simulink model "Fuzzy_manobra_aplicado_2015b"  (R2015b)
settings: Solver=ode1  StartTime=0.0  StopTime=t_final  FixedStep=0.01  RelTol=1e-3
values from neighbouring files (symbols this model uses):
  fis = readfis(['CONTROLADORES/' controlador '.fis'])    [inicia_fuzzy_manobra.m]
  k_i = 1    [inicia_fuzzy_manobra.m]
  k_p = 2.5    [inicia_fuzzy_manobra.m]
  L = 0.1175    [inicia_fuzzy_manobra.m]
  N_sp = size(setpoints,1)    [inicia_fuzzy_manobra.m]
  R = 0.034    [inicia_fuzzy_manobra.m]
undefined symbols (not defined in the file or in its folder): HIL, magnitude, setpoints
libraries: quarc_library x6, simulink x3, fuzblock x1
settings Model: SimulationMode=external  ExtModeTrigDuration=10000  Creator=rhuq  LastModifiedBy=LabMTrônica01
settings SolverCC: PositivePriorityOrder=on
settings DataIOCC: LimitDataPoints=off  SaveFormat=Array  SignalLoggingSaveFormat=ModelDataLogs
settings OptimizationCC: ExpressionDepthLimit=2147483647  InitFltsAndDblsToZero=on
settings DebuggingCC: SaveWithParameterizedLinksMsg=none  UnderspecifiedInitializationDetection=Classic  MergeDetectMultiDrivingBlocksExec=none  SolverPrmCheckMsg=warning  ParameterPrecisionLossMsg=none  FcnCallInpInsideContextMsg=EnableAllAsWarning  StateNameClashWarn=warning
settings HardwareCC: ProdBitPerPointer=32  ProdLargestAtomicFloat=None  ProdIntDivRoundTo=Undefined  ProdEndianess=Unspecified  ProdWordSize=32  ProdHWDeviceType=32-bit Generic
settings SFSimCC: SimParseCustomCode=off
settings RTWCC: SystemTargetFile=quarc_linux_duovero.tlc  TemplateMakefile=quarc_default_tmf  Description=QUARC Linux DuoVero Target
settings STFCustomTargetCC: TargetLibSuffix=.a  TargetPreCompLibLocation=C:\PROGRA~3\QUARC\lib\2015b\LINUX_~1\release  GeneratePreprocessorConditionals=Use local settings  CombineOutputUpdateFcns=on  GRTInterface=off  SystemTargetFile=quarc_linux_duovero.tlc
settings GRTTargetCC: TargetLibSuffix=.a  TargetPreCompLibLocation=C:\PROGRA~3\QUARC\lib\2015b\LINUX_~1\release  ParMdlRefBuildCompliant=off  CompOptLevelCompliant=off  MatFileLogging=off  UseToolchainInfoCompliant=off  ExtMode=on  ExtModeMexFile=quarc_comm  ExtModeMexArgs='-w -d /tmp -uri %u'
settings ConfigComp: CovModelRefEnable=Off

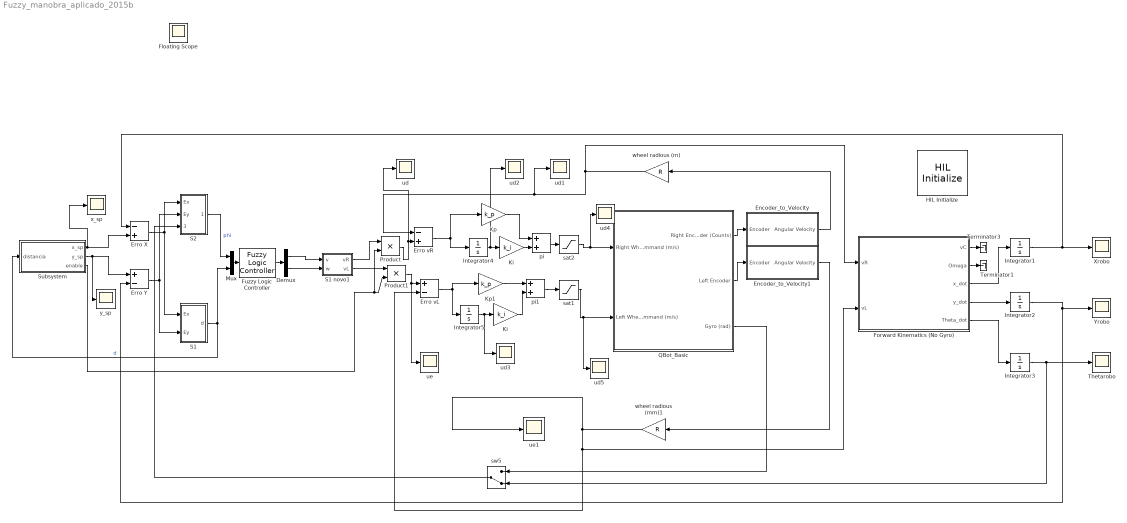
== system Fuzzy_manobra_aplicado_2015b ==
  Demux : Demux  Outputs=2
  Encoder_to_Velocity : Subsystem
  Encoder_to_Velocity1 : Subsystem
  Erro X : Sum  Inputs=-+
  Erro Y : Sum  Inputs=+-
  Erro vL : Sum  Inputs=+-
  Erro vR : Sum  Inputs=-+
  Forward Kinematics (No Gyro) : Subsystem
  Fuzzy Logic Controller : fuzblock/Fuzzy Logic  Controller  fis=[fis]
  HIL Initialize : quarc_library/Data Acquisition/Generic/Configuration/HIL Initialize  Priority=-99  object_name=HIL-1  board_type=qbot2  board_number=0  board_options=enc0_dir=0;enc0_filter=1;enc0_a=0;enc0_b=0;enc0_z=1;enc0_reload=0;enc1_dir=0;enc1_filter=1;enc1_a=0;enc1_b=0;enc1_z=1;enc1_reload=0;pwm0_immediate=0;pwm1_immediate=0;pwm2_immediate=0;pwm3_immediate=0;  exclusive=off  active=off  hardware_clocks=[]  clock_modes=[]  initial_clock_frequencies=[]  set_clock_params_at_start=off  set_clock_params_at_switch_in=off  set_clock_frequencies_at_start=off  set_clock_frequencies_at_switch_in=off  analog_input_channels=[0:9]  analog_input_maximums=[5 5 5 5 16.5 3.3 3.3 3.3 3.3]  analog_input_minimums=[0 0 0 0 0 0 0 0 0]  set_analog_input_params_at_start=off  set_analog_input_params_at_switch_in=off  analog_output_channels=[]  analog_output_maximums=[]  analog_output_minimums=[]  initial_analog_outputs=[]  final_analog_outputs=[]  watchdog_analog_outputs=[]  set_analog_output_params_at_start=off  set_analog_output_params_at_switch_in=off  set_analog_outputs_at_start=off  set_analog_outputs_at_switch_in=off  set_analog_outputs_at_terminate=off  set_analog_outputs_at_switch_out=off  set_analog_outputs_on_watchdog=off  digital_input_channels=[]  digital_output_channels=[]  digital_output_configuration=[]  initial_digital_outputs=[0]  final_digital_outputs=[0]  watchdog_digital_outputs=[0]  set_digital_output_params_at_start=off  set_digital_output_params_at_switch_in=off  set_digital_outputs_at_start=on  set_digital_outputs_at_switch_in=off  set_digital_outputs_at_terminate=on  set_digital_outputs_at_switch_out=off  set_digital_outputs_on_watchdog=on  encoder_channels=[0:3]  quadrature=[4]  encoder_filter_frequency=[]  initial_encoder_counts=[0]  set_encoder_params_at_start=on  set_encoder_params_at_switch_in=off  set_encoder_counts_at_start=on  set_encoder_counts_at_switch_in=off  pwm_channels=[0:3]  pwm_modes=[0 0 0 0]  pwm_frequency=[20e6/1024 20e6/1024 20e6/1024 20e6/1024]  pwm_configuration=[0]  pwm_alignment=[0]  pwm_polarity=[1]  pwm_leading_deadband=[0]  pwm_trailing_deadband=[0]  initial_pwm_outputs=[0]  final_pwm_outputs=[0]  watchdog_pwm_outputs=[0]  set_pwm_params_at_start=on  set_pwm_params_at_switch_in=off  set_pwm_outputs_at_start=on  set_pwm_outputs_at_switch_in=off  set_pwm_outputs_at_terminate=on  set_pwm_outputs_at_switch_out=off  set_pwm_outputs_on_watchdog=on  other_output_channels=[2000:2001]  initial_other_outputs=[0 0 7]  final_other_outputs=[0 0 1]  watchdog_other_outputs=[]  set_other_outputs_at_start=on  set_other_outputs_at_switch_in=off  set_other_outputs_at_terminate=on  set_other_outputs_at_switch_out=off  set_other_outputs_on_watchdog=off
  Integrator1 : Integrator  ContinuousStateAttributes='x_a'
  Integrator2 : Integrator  ContinuousStateAttributes='y_a'
  Integrator3 : Integrator  ContinuousStateAttributes='theta'
  Integrator4 : Integrator  ContinuousStateAttributes='ePI_d'
  Integrator5 : Integrator  ContinuousStateAttributes='ePI_e'
  Ki : Gain  Gain=k_i
  "Ki " : Gain  Gain=k_i
  Kp : Gain  Gain=k_p
  Kp1 : Gain  Gain=k_p
  Mux : Mux  Inputs=2
  Product : Product
  Product1 : Product
  QBot_Basic : Subsystem
  S1 : Subsystem
  S1 novo1 : Subsystem
  S2 : Subsystem
  Subsystem : Subsystem
  Terminator1 : Terminator
  Terminator3 : Terminator
  Thetarobo : Scope
  Xrobo : Scope
  Yrobo : Scope
  pi : Sum
  pi1 : Sum
  sat1 : Saturate  UpperLimit=0.65  LowerLimit=-0.65
  sat2 : Saturate  UpperLimit=0.65  LowerLimit=-0.65
  sw5 : ManualSwitch  CurrentSetting=0
  ud{,1..5} (6 alike) : Scope
  ue : Scope
  ue1 : Scope
  wheel radious (m) : Gain  Gain=R
  wheel radious (mm)1 : Gain  Gain=R
  x_sp : Scope
  y_sp : Scope
  Floating Scope : Scope
  wires:
  QBot_Basic/1(Right Encoder (Counts)) -> Encoder_to_Velocity/1(Encoder)
  QBot_Basic/2(Left Encoder) -> Encoder_to_Velocity1/1(Encoder)
  Erro X/1 -> S1/1(Ex), S2/1(Ex)
  Erro Y/1 -> S1/2(Ey), S2/2(Ey)
  Mux/1 -> Fuzzy Logic Controller/1
  S2/1(phi) -> Mux/1  "phi"
  Subsystem/2(y_sp) -> Erro Y/1, y_sp/1
  Subsystem/1(x_sp) -> x_sp/1, Erro X/2
  Fuzzy Logic Controller/1 -> Demux/1
  S1 novo1/2(vL) -> Product1/1
  Encoder_to_Velocity1/1(Angular Velocity) -> wheel radious (mm)1/1
  Integrator2/1 -> Yrobo/1, Erro Y/2
  S1/1(d) -> Mux/2, Subsystem/1("distancia ")  "d"
  Demux/1 -> S1 novo1/1(v)
  Demux/2 -> S1 novo1/2(w)
  Encoder_to_Velocity/1(Angular Velocity) -> wheel radious (m)/1
  Forward Kinematics (No Gyro)/3(x_dot) -> Integrator1/1
  Forward Kinematics (No Gyro)/4(y_dot) -> Integrator2/1
  Forward Kinematics (No Gyro)/5(Theta_dot) -> Integrator3/1
  Integrator1/1 -> Xrobo/1, Erro X/1
  Integrator3/1 -> Thetarobo/1, sw5/2
  wheel radious (m)/1 -> ud1/1, Erro vR/1, Forward Kinematics (No Gyro)/1(vR)
  wheel radious (mm)1/1 -> Erro vL/2, Forward Kinematics (No Gyro)/2(vL), ue1/1
  Erro vR/1 -> Kp/1, Integrator4/1
  sw5/1 -> S2/3(theta)
  QBot_Basic/3(Gyro (rad)) -> sw5/1
  Subsystem/3(enable) -> Product/2, Product1/2
  S1 novo1/1(vR) -> Product/1
  Product/1 -> ud/1, Erro vR/2
  sat1/1 -> ud5/1, QBot_Basic/2(Left Wheel Command (m/s))
  sat2/1 -> ud4/1, QBot_Basic/1(Right Wheel Command (m/s))
  Forward Kinematics (No Gyro)/1(vC) -> Terminator3/1
  Forward Kinematics (No Gyro)/2(Omega) -> Terminator1/1
  Erro vL/1 -> Kp1/1, Integrator5/1
  Integrator5/1 -> ud3/1, Ki/1
  Integrator4/1 -> ud2/1, "Ki "/1
  pi1/1 -> sat1/1
  "Ki "/1 -> pi/2
  pi/1 -> sat2/1
  Kp/1 -> pi/1
  Kp1/1 -> pi1/1
  Ki/1 -> pi1/2
  Product1/1 -> ue/1, Erro vL/1

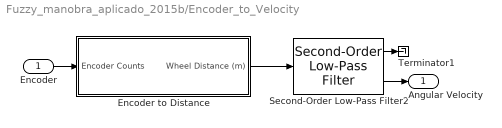
== system Fuzzy_manobra_aplicado_2015b/Encoder_to_Velocity ==
  Encoder : Inport
  Encoder to Distance : Subsystem
  Second-Order Low-Pass Filter2 : quarc_library/Continuous/Second-Order Low-Pass Filter  params_source=Internal (dialog parameters)  input_width=10  input_zeta=1  input_init=0
  Terminator1 : Terminator
  Angular Velocity : Outport
  wires:
  Second-Order Low-Pass Filter2/2 -> Angular Velocity/1
  Encoder/1 -> Encoder to Distance/1(Encoder Counts)
  Encoder to Distance/1(Wheel Distance (m)) -> Second-Order Low-Pass Filter2/1
  Second-Order Low-Pass Filter2/1 -> Terminator1/1

== system Fuzzy_manobra_aplicado_2015b/Encoder_to_Velocity1 ==
  Encoder : Inport
  Encoder to Distance : Subsystem
  Second-Order Low-Pass Filter2 : quarc_library/Continuous/Second-Order Low-Pass Filter  params_source=Internal (dialog parameters)  input_width=10  input_zeta=1  input_init=0
  Terminator1 : Terminator
  Angular Velocity : Outport
  wires:
  Second-Order Low-Pass Filter2/1 -> Terminator1/1
  Encoder to Distance/1(Wheel Distance (m)) -> Second-Order Low-Pass Filter2/1
  Encoder/1 -> Encoder to Distance/1(Encoder Counts)
  Second-Order Low-Pass Filter2/2 -> Angular Velocity/1

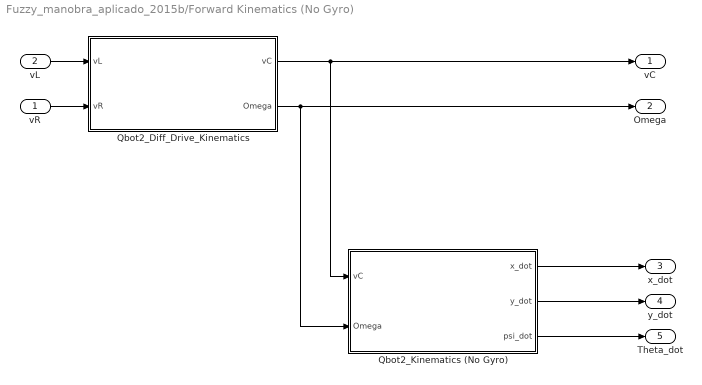
== system Fuzzy_manobra_aplicado_2015b/Forward Kinematics (No Gyro) ==
  vR : Inport
  vL : Inport  Port=2
  Qbot2_Diff_Drive_Kinematics : Subsystem
  Qbot2_Kinematics (No Gyro) : Subsystem
  vC : Outport
  Omega : Outport  Port=2
  x_dot : Outport  Port=3
  y_dot : Outport  Port=4
  Theta_dot : Outport  Port=5
  wires:
  Qbot2_Diff_Drive_Kinematics/2(Omega) -> Qbot2_Kinematics (No Gyro)/2(Omega), Omega/1
  vR/1 -> Qbot2_Diff_Drive_Kinematics/2(vR)
  vL/1 -> Qbot2_Diff_Drive_Kinematics/1(vL)
  Qbot2_Diff_Drive_Kinematics/1(vC) -> Qbot2_Kinematics (No Gyro)/1(vC), vC/1
  Qbot2_Kinematics (No Gyro)/2(y_dot) -> y_dot/1
  Qbot2_Kinematics (No Gyro)/1(x_dot) -> x_dot/1
  Qbot2_Kinematics (No Gyro)/3(psi_dot) -> Theta_dot/1

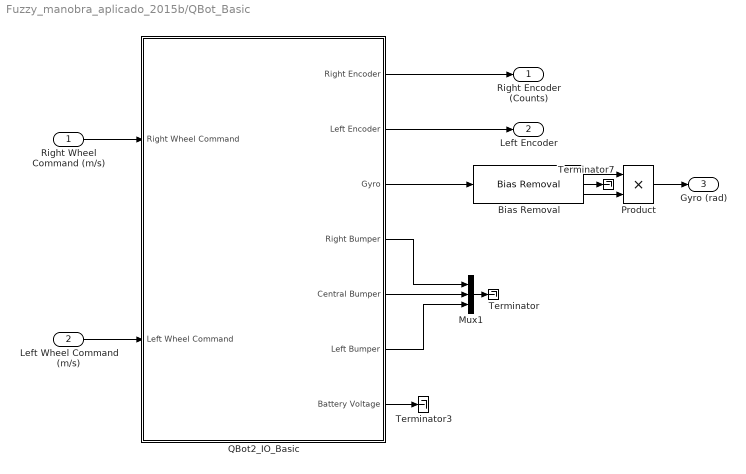
== system Fuzzy_manobra_aplicado_2015b/QBot_Basic ==
  Right Wheel Command (m/s) : Inport
  Left Wheel Command (m/s) : Inport  Port=2
  Bias Removal : quarc_library/Discrete/Bias Removal  start_time=3  end_time=4  switch_id=0  sample_time=qc_get_step_size
  Mux1 : Mux  Inputs=3
  Product : Product  RndMeth=Zero
  QBot2_IO_Basic : Subsystem
  Terminator : Terminator
  Terminator3 : Terminator
  Terminator7 : Terminator
  Right Encoder (Counts) : Outport
  Left Encoder : Outport  Port=2
  Gyro (rad) : Outport  Port=3
  wires:
  Mux1/1 -> Terminator/1
  QBot2_IO_Basic/3(Gyro) -> Bias Removal/1
  Product/1 -> Gyro (rad)/1
  Bias Removal/3 -> Product/2
  Bias Removal/1 -> Product/1
  Bias Removal/2 -> Terminator7/1
  QBot2_IO_Basic/2(Left Encoder) -> Left Encoder/1
  QBot2_IO_Basic/1(Right Encoder) -> Right Encoder (Counts)/1
  Left Wheel Command (m/s)/1 -> QBot2_IO_Basic/2(Left Wheel Command)
  Right Wheel Command (m/s)/1 -> QBot2_IO_Basic/1(Right Wheel Command)
  QBot2_IO_Basic/6(Left Bumper) -> Mux1/3
  QBot2_IO_Basic/5(Central Bumper) -> Mux1/2
  QBot2_IO_Basic/4(Right Bumper) -> Mux1/1
  QBot2_IO_Basic/7(Battery Voltage) -> Terminator3/1

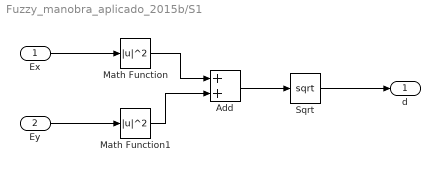
== system Fuzzy_manobra_aplicado_2015b/S1 ==
  Ex : Inport
  Ey : Inport  Port=2
  Add : Sum
  Math Function : Math  Operator=magnitude^2  SaturateOnIntegerOverflow=on
  Math Function1 : Math  Operator=magnitude^2  SaturateOnIntegerOverflow=on
  Sqrt : Sqrt  SaturateOnIntegerOverflow=on
  d : Outport
  wires:
  Math Function/1 -> Add/1
  Ey/1 -> Math Function1/1
  Add/1 -> Sqrt/1
  Ex/1 -> Math Function/1
  Sqrt/1 -> d/1
  Math Function1/1 -> Add/2

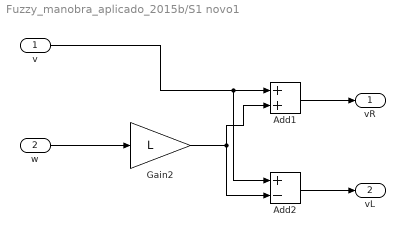
== system Fuzzy_manobra_aplicado_2015b/S1 novo1 ==
  v : Inport
  w : Inport  Port=2
  Add1 : Sum
  Add2 : Sum  Inputs=+-
  Gain2 : Gain  Gain=L
  vR : Outport
  vL : Outport  Port=2
  wires:
  Add1/1 -> vR/1
  v/1 -> Add2/1, Add1/1
  Gain2/1 -> Add1/2, Add2/2
  w/1 -> Gain2/1
  Add2/1 -> vL/1

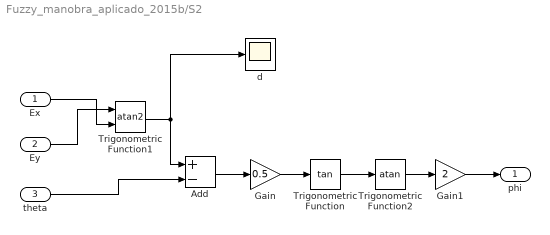
== system Fuzzy_manobra_aplicado_2015b/S2 ==
  Ex : Inport
  Ey : Inport  Port=2
  theta : Inport  Port=3
  Add : Sum  Inputs=+-
  Gain : Gain  Gain=0.5
  Gain1 : Gain  Gain=2
  Trigonometric Function : Trigonometry  Operator=tan
  Trigonometric Function1 : Trigonometry  Operator=atan2
  Trigonometric Function2 : Trigonometry  Operator=atan
  d : Scope
  phi : Outport
  wires:
  Ey/1 -> Trigonometric Function1/1
  Ex/1 -> Trigonometric Function1/2
  Trigonometric Function1/1 -> Add/1, d/1
  theta/1 -> Add/2
  Trigonometric Function/1 -> Trigonometric Function2/1
  Trigonometric Function2/1 -> Gain1/1
  Gain/1 -> Trigonometric Function/1
  Gain1/1 -> phi/1
  Add/1 -> Gain/1

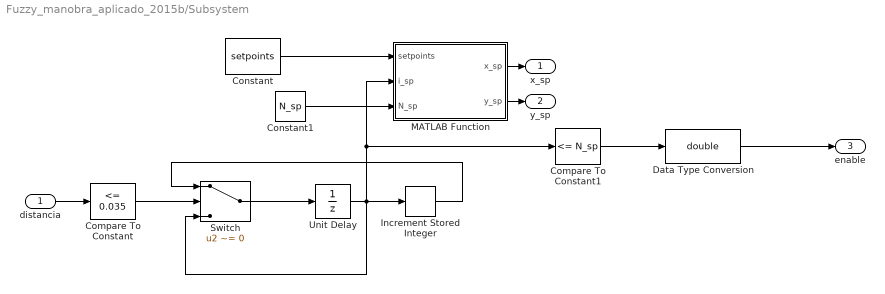
== system Fuzzy_manobra_aplicado_2015b/Subsystem ==
  "distancia " : Inport
  Compare To Constant : simulink/Logic and Bit Operations/Compare To Constant  relop=<=  const=0.035  OutDataTypeStr=boolean
  Compare To Constant1 : simulink/Logic and Bit Operations/Compare To Constant  relop=<=  const=N_sp  OutDataTypeStr=boolean
  Constant : Constant  Value=setpoints  VectorParams1D=off
  Constant1 : Constant  Value=N_sp
  Data Type Conversion : DataTypeConversion  OutDataTypeStr=double
  Increment Stored Integer : simulink/Additional Math & Discrete/Additional Math: Increment - Decrement/Increment Stored Integer
  MATLAB Function : MATLAB Function  TreatAsAtomicUnit=on
  Switch : Switch  Criteria=u2 ~= 0
  Unit Delay : UnitDelay  InitialCondition=1  SampleTime=-1
  x_sp : Outport
  y_sp : Outport  Port=2
  enable : Outport  Port=3
  wires:
  Constant/1 -> MATLAB Function/1(setpoints)
  Constant1/1 -> MATLAB Function/3(N_sp)
  Compare To Constant/1 -> Switch/2
  "distancia "/1 -> Compare To Constant/1
  Switch/1 -> Unit Delay/1
  Unit Delay/1 -> MATLAB Function/2(i_sp), Compare To Constant1/1, Increment Stored Integer/1, Switch/3
  Increment Stored Integer/1 -> Switch/1
  MATLAB Function/1(x_sp) -> x_sp/1
  MATLAB Function/2(y_sp) -> y_sp/1
  Compare To Constant1/1 -> Data Type Conversion/1
  Data Type Conversion/1 -> enable/1

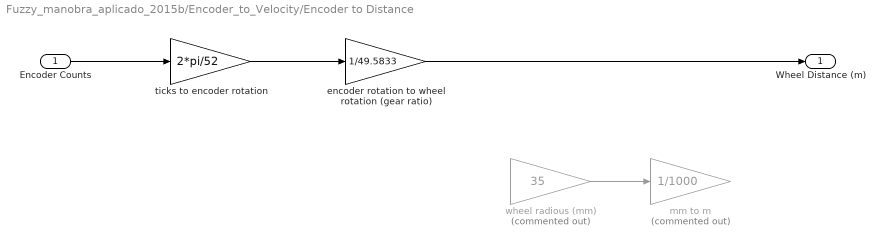
== system Fuzzy_manobra_aplicado_2015b/Encoder_to_Velocity/Encoder to Distance ==
  Encoder Counts : Inport
  " encoder rotation to wheel rotation (gear ratio)" : Gain  Gain=1/49.5833
  mm to m : Gain  Commented=on  Gain=1/1000
  ticks to encoder rotation : Gain  Gain=2*pi/52
  wheel radious (mm) : Gain  Commented=on  Gain=35
  Wheel Distance (m) : Outport
  wires:
  ticks to encoder rotation/1 -> " encoder rotation to wheel rotation (gear ratio)"/1
  Encoder Counts/1 -> ticks to encoder rotation/1
  " encoder rotation to wheel rotation (gear ratio)"/1 -> Wheel Distance (m)/1
  wheel radious (mm)/1 -> mm to m/1

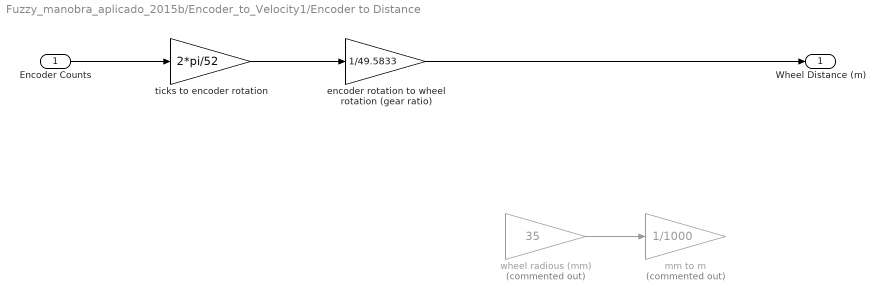
== system Fuzzy_manobra_aplicado_2015b/Encoder_to_Velocity1/Encoder to Distance ==
  Encoder Counts : Inport
  " encoder rotation to wheel rotation (gear ratio)" : Gain  Gain=1/49.5833
  mm to m : Gain  Commented=on  Gain=1/1000
  ticks to encoder rotation : Gain  Gain=2*pi/52
  wheel radious (mm) : Gain  Commented=on  Gain=35
  Wheel Distance (m) : Outport
  wires:
  Encoder Counts/1 -> ticks to encoder rotation/1
  ticks to encoder rotation/1 -> " encoder rotation to wheel rotation (gear ratio)"/1
  " encoder rotation to wheel rotation (gear ratio)"/1 -> Wheel Distance (m)/1
  wheel radious (mm)/1 -> mm to m/1

== system Fuzzy_manobra_aplicado_2015b/Forward Kinematics (No Gyro)/Qbot2_Diff_Drive_Kinematics ==
  vL : Inport
  vR : Inport  Port=2
  Qbot2_Diff_Drive_Kinematics : MATLAB Function  TreatAsAtomicUnit=on
  vC : Outport
  Omega : Outport  Port=2
  wires:
  vL/1 -> Qbot2_Diff_Drive_Kinematics/1(vL)
  Qbot2_Diff_Drive_Kinematics/1(vC) -> vC/1
  vR/1 -> Qbot2_Diff_Drive_Kinematics/2(vR)
  Qbot2_Diff_Drive_Kinematics/2(Omega) -> Omega/1

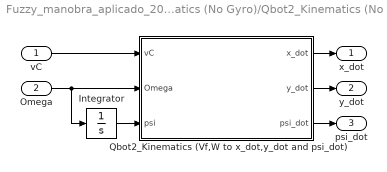
== system Fuzzy_manobra_aplicado_2015b/Forward Kinematics (No Gyro)/Qbot2_Kinematics (No Gyro) ==
  vC : Inport
  Omega : Inport  Port=2
  Integrator : Integrator
  Qbot2_Kinematics (Vf,W to x_dot,y_dot and psi_dot) : MATLAB Function  TreatAsAtomicUnit=on
  x_dot : Outport
  y_dot : Outport  Port=2
  psi_dot : Outport  Port=3
  wires:
  Qbot2_Kinematics (Vf,W to x_dot,y_dot and psi_dot)/3(psi_dot) -> psi_dot/1
  Integrator/1 -> Qbot2_Kinematics (Vf,W to x_dot,y_dot and psi_dot)/3(psi)
  vC/1 -> Qbot2_Kinematics (Vf,W to x_dot,y_dot and psi_dot)/1(vC)
  Qbot2_Kinematics (Vf,W to x_dot,y_dot and psi_dot)/1(x_dot) -> x_dot/1
  Omega/1 -> Integrator/1, Qbot2_Kinematics (Vf,W to x_dot,y_dot and psi_dot)/2(Omega)
  Qbot2_Kinematics (Vf,W to x_dot,y_dot and psi_dot)/2(y_dot) -> y_dot/1

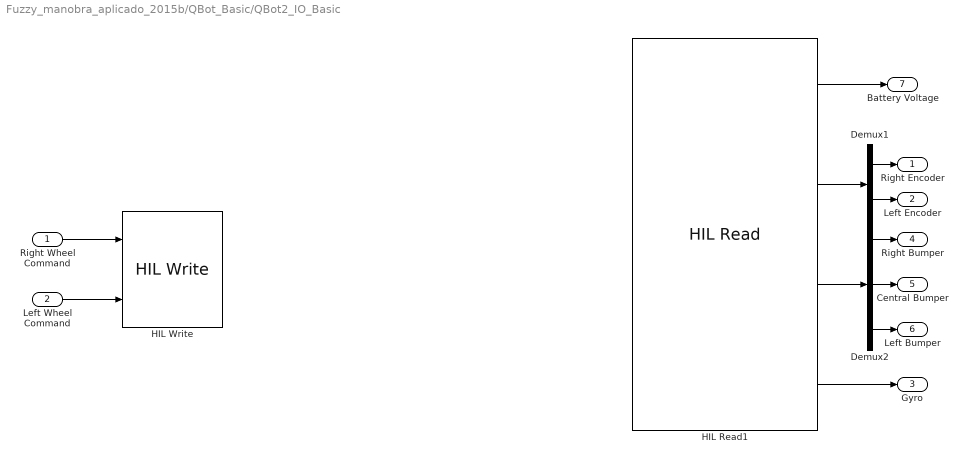
== system Fuzzy_manobra_aplicado_2015b/QBot_Basic/QBot2_IO_Basic ==
  Right Wheel Command : Inport
  Left Wheel Command : Inport  Port=2
  Demux1 : Demux  Outputs=2
  Demux2 : Demux  Outputs=3
  HIL Read1 : quarc_library/Data Acquisition/Generic/Immediate I//O/HIL Read  object_name=HIL-1  analog_channels=[4]  encoder_channels=[2 3]  digital_channels=[8 9 10]  other_channels=[1002]  sample_time=qc_get_step_size  active=on  vector_output=on  data_type_mode=Inherit via back propagation  encoder_data_type=double  digital_data_type=boolean
  HIL Write : quarc_library/Data Acquisition/Generic/Immediate I//O/HIL Write  object_name=HIL-1  analog_channels=[]  pwm_channels=[]  digital_channels=[]  other_channels=[2000:2001]  sample_time=-1  active=on  vector_input=off
  Right Encoder : Outport
  Left Encoder : Outport  Port=2
  Gyro : Outport  Port=3
  Right Bumper : Outport  Port=4
  Central Bumper : Outport  Port=5
  Left Bumper : Outport  Port=6
  Battery Voltage : Outport  Port=7
  wires:
  Demux2/3 -> Left Bumper/1
  Demux2/2 -> Central Bumper/1
  Demux2/1 -> Right Bumper/1
  HIL Read1/2 -> Demux1/1
  Left Wheel Command/1 -> HIL Write/2
  Right Wheel Command/1 -> HIL Write/1
  Demux1/2 -> Left Encoder/1
  Demux1/1 -> Right Encoder/1
  HIL Read1/4 -> Gyro/1
  HIL Read1/3 -> Demux2/1
  HIL Read1/1 -> Battery Voltage/1

== matlab function Fuzzy_manobra_aplicado_2015b/Forward Kinematics (No Gyro)/Qbot2_Diff_Drive_Kinematics/Qbot2_Diff_Drive_Kinematics ==
  data: vL input; vC output; vR input; Omega output
function [vC,Omega] = fcn(vL,vR)
%#codegen

d= 0.235;

vC=0.5*(vL+vR);
Omega=(1/d)*(vR-vL);

== matlab function Fuzzy_manobra_aplicado_2015b/Subsystem/MATLAB Function ==
  data: setpoints input; x_sp output; i_sp input; N_sp input; y_sp output
function [x_sp, y_sp] = fcn(setpoints,i_sp,N_sp)
%#codegen
if i_sp<1 || isempty(i_sp)
    i_sp = 1;
end
i_sp = int64(i_sp);
if i_sp<=N_sp
    x_sp = setpoints(i_sp,1);
    y_sp = setpoints(i_sp,2);
else
    x_sp = setpoints(end,1);
    y_sp = setpoints(end,2);
end
end

== matlab function Fuzzy_manobra_aplicado_2015b/Forward Kinematics (No Gyro)/Qbot2_Kinematics (No Gyro)/Qbot2_Kinematics (Vf,W to x_dot,y_dot and psi_dot) ==
  data: vC input; x_dot output; Omega input; y_dot output; psi input; psi_dot output
function [x_dot,y_dot,psi_dot] = fcn(vC,Omega,psi)
%#codegen


x_dot=cos(psi)*vC;
y_dot=sin(psi)*vC;
psi_dot= Omega;
